simulink model "pole_placement_disturbance"  (R2017a)
settings: Solver=VariableStepAuto  StartTime=0.0  StopTime=10  RelTol=1e-3
values from neighbouring files (symbols this model uses):
  DCgain5 = D5d + C5cl*inv(eye(3)-A5cl)*B5d    [q13.m]    (also in q5.m; q5_reduced.m)
  h5 = 2.5*pi/w    [q13.m]    (also in q5.m = 2*pi/w; q5_reduced.m = 2*pi/w)
  K5_discr = place(A5d, B5d, P_discr)    [q13.m]    (also in q5.m; q5_reduced.m)
undefined symbols (not defined in the file or in its folder): A5d, B5d, C5d, D5d
settings Model: Creator=Aleksandra  LastModifiedBy=Aleksandra

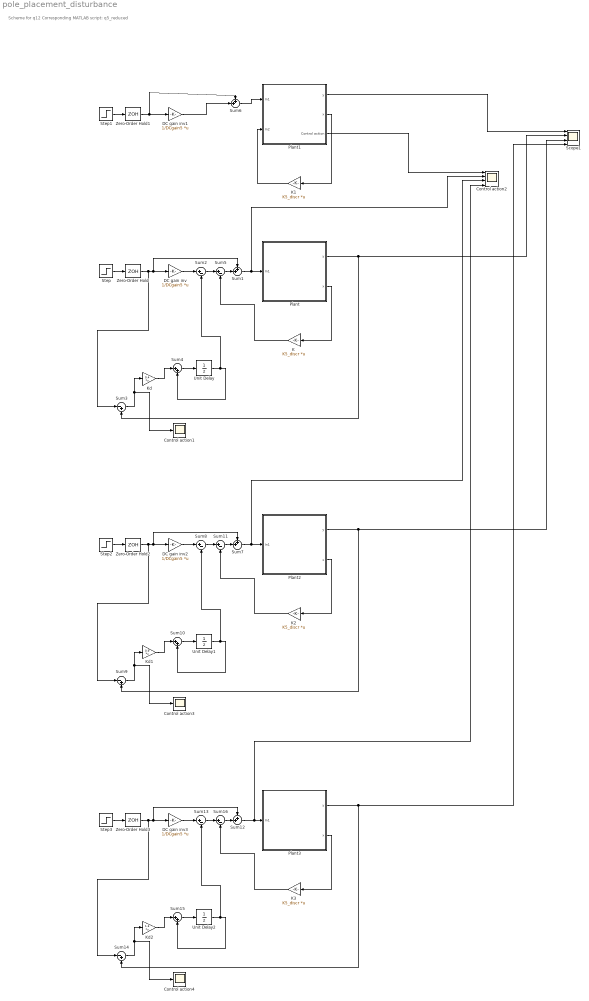
== system pole_placement_disturbance ==
  note: Scheme for q12
      | Corresponding MATLAB script: q5_reduced
  Control action1 : Scope
  Control action2 : Scope  NumInputPorts=4
  Control action3 : Scope
  Control action4 : Scope
  DC gain inv{,1..3} (4 alike) : Gain  Gain=1/DCgain5  Multiplication=Matrix(K*u)
  K{,1..3} (4 alike) : Gain  Gain=K5_discr  Multiplication=Matrix(K*u)
  Kd : Gain  Gain=0.4  Multiplication=Matrix(K*u)
  Kd1 : Gain  Gain=0.9  Multiplication=Matrix(K*u)
  Kd2 : Gain  Gain=1.3  Multiplication=Matrix(K*u)
  Plant : Subsystem
  Plant1 : Subsystem
  Plant2 : Subsystem
  Plant3 : Subsystem
  Scope1 : Scope  NumInputPorts=4
  Step{,1..3} (4 alike) : Step  Time=0  SampleTime=0
  Sum{1,6..7,12} (4 alike) : Sum  Inputs=++|
  Sum10 : Sum  Inputs=|++
  Sum{2,5,8,11,13,16} (6 alike) : Sum  Inputs=|+-
  Sum14 : Sum  Inputs=|-+
  Sum15 : Sum  Inputs=|++
  Sum3 : Sum  Inputs=|-+
  Sum4 : Sum  Inputs=|++
  Sum9 : Sum  Inputs=|-+
  Unit Delay : UnitDelay  SampleTime=-1
  Unit Delay1 : UnitDelay  SampleTime=-1
  Unit Delay2 : UnitDelay  SampleTime=-1
  Zero-Order Hold{,1..3} (4 alike) : ZeroOrderHold  SampleTime=h5
  wires:
  Step/1 -> Zero-Order Hold/1
  Plant/1(y) -> Sum3/2, Scope1/2
  Plant/2(x) -> K/1
  K/1 -> Sum5/2
  Zero-Order Hold/1 -> Sum3/1, Sum1/1, DC gain inv/1
  DC gain inv/1 -> Sum2/1
  Sum1/1 -> Control action2/2, Plant/1(In1)
  Sum2/1 -> Sum5/1
  Sum3/1 -> Control action1/1, Kd/1
  Sum4/1 -> Unit Delay/1
  Kd/1 -> Sum4/1
  Unit Delay/1 -> Sum2/2, Sum4/2
  Sum5/1 -> Sum1/2
  DC gain inv1/1 -> Sum6/2
  Plant1/3(Control action) -> Control action2/1
  Zero-Order Hold1/1 -> Sum6/1, DC gain inv1/1
  Plant1/1(y) -> Scope1/1
  K1/1 -> Plant1/2(In2)
  Plant1/2(x) -> K1/1
  Step1/1 -> Zero-Order Hold1/1
  Sum6/1 -> Plant1/1(In1)
  Zero-Order Hold2/1 -> Sum9/1, Sum7/1, DC gain inv2/1
  Plant2/1(y) -> Scope1/3, Sum9/2
  Step2/1 -> Zero-Order Hold2/1
  Sum10/1 -> Unit Delay1/1
  Sum11/1 -> Sum7/2
  Unit Delay1/1 -> Sum8/2, Sum10/2
  Sum7/1 -> Control action2/3, Plant2/1(In1)
  Plant2/2(x) -> K2/1
  Sum8/1 -> Sum11/1
  Kd1/1 -> Sum10/1
  K2/1 -> Sum11/2
  Sum9/1 -> Control action3/1, Kd1/1
  DC gain inv2/1 -> Sum8/1
  Zero-Order Hold3/1 -> Sum14/1, Sum12/1, DC gain inv3/1
  Plant3/1(y) -> Scope1/4, Sum14/2
  Step3/1 -> Zero-Order Hold3/1
  Sum15/1 -> Unit Delay2/1
  Sum16/1 -> Sum12/2
  Unit Delay2/1 -> Sum13/2, Sum15/2
  Sum12/1 -> Control action2/4, Plant3/1(In1)
  Plant3/2(x) -> K3/1
  Sum13/1 -> Sum16/1
  Kd2/1 -> Sum15/1
  K3/1 -> Sum16/2
  Sum14/1 -> Control action4/1, Kd2/1
  DC gain inv3/1 -> Sum13/1

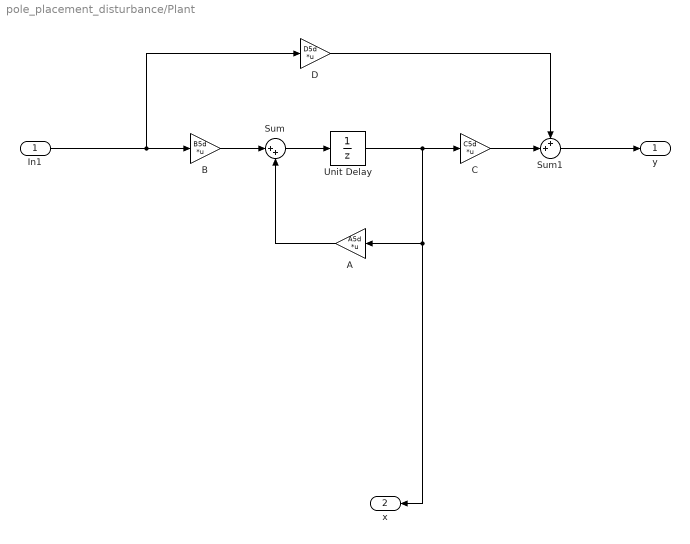
== system pole_placement_disturbance/Plant ==
  In1 : Inport
  A : Gain  Gain=A5d  Multiplication=Matrix(K*u)
  B : Gain  Gain=B5d  Multiplication=Matrix(K*u)
  C : Gain  Gain=C5d  Multiplication=Matrix(K*u)
  D : Gain  Gain=D5d  Multiplication=Matrix(K*u)
  Sum : Sum  Inputs=|++
  Sum1 : Sum  Inputs=++|
  Unit Delay : UnitDelay  SampleTime=-1
  y : Outport
  x : Outport  Port=2
  wires:
  Sum/1 -> Unit Delay/1
  A/1 -> Sum/2
  D/1 -> Sum1/1
  C/1 -> Sum1/2
  Sum1/1 -> y/1
  B/1 -> Sum/1
  In1/1 -> D/1, B/1
  Unit Delay/1 -> x/1, A/1, C/1

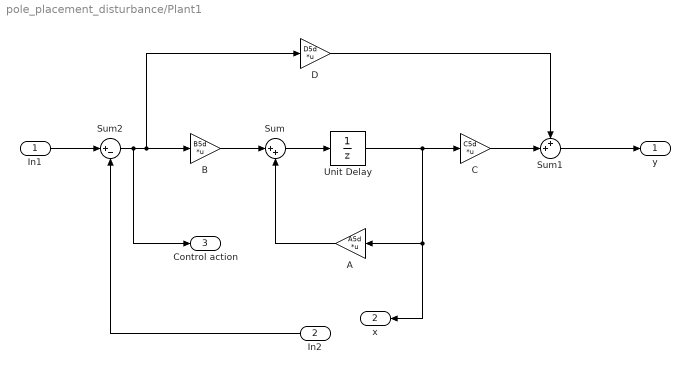
== system pole_placement_disturbance/Plant1 ==
  In1 : Inport
  In2 : Inport  Port=2
  A : Gain  Gain=A5d  Multiplication=Matrix(K*u)
  B : Gain  Gain=B5d  Multiplication=Matrix(K*u)
  C : Gain  Gain=C5d  Multiplication=Matrix(K*u)
  D : Gain  Gain=D5d  Multiplication=Matrix(K*u)
  Sum : Sum  Inputs=|++
  Sum1 : Sum  Inputs=++|
  Sum2 : Sum  Inputs=|+-
  Unit Delay : UnitDelay  SampleTime=-1
  y : Outport
  x : Outport  Port=2
  Control action : Outport  Port=3
  wires:
  Sum/1 -> Unit Delay/1
  A/1 -> Sum/2
  D/1 -> Sum1/1
  C/1 -> Sum1/2
  Sum1/1 -> y/1
  B/1 -> Sum/1
  Sum2/1 -> Control action/1, D/1, B/1
  Unit Delay/1 -> x/1, A/1, C/1
  In2/1 -> Sum2/2
  In1/1 -> Sum2/1

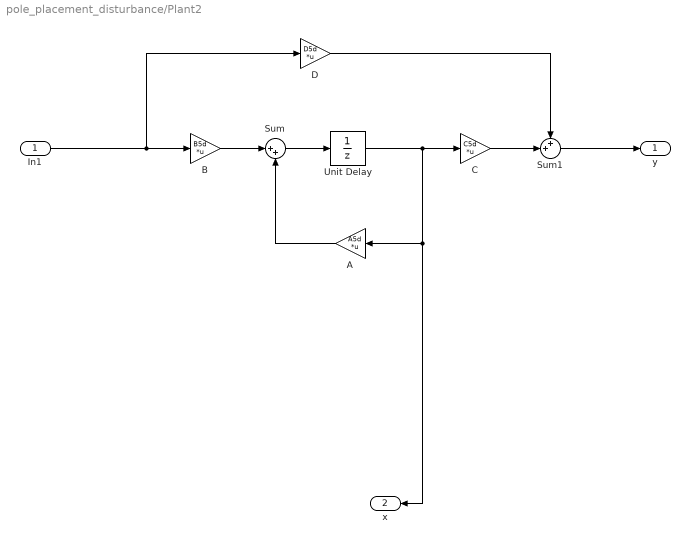
== system pole_placement_disturbance/Plant2 ==
  In1 : Inport
  A : Gain  Gain=A5d  Multiplication=Matrix(K*u)
  B : Gain  Gain=B5d  Multiplication=Matrix(K*u)
  C : Gain  Gain=C5d  Multiplication=Matrix(K*u)
  D : Gain  Gain=D5d  Multiplication=Matrix(K*u)
  Sum : Sum  Inputs=|++
  Sum1 : Sum  Inputs=++|
  Unit Delay : UnitDelay  SampleTime=-1
  y : Outport
  x : Outport  Port=2
  wires:
  Sum/1 -> Unit Delay/1
  A/1 -> Sum/2
  D/1 -> Sum1/1
  C/1 -> Sum1/2
  Sum1/1 -> y/1
  B/1 -> Sum/1
  In1/1 -> D/1, B/1
  Unit Delay/1 -> x/1, A/1, C/1

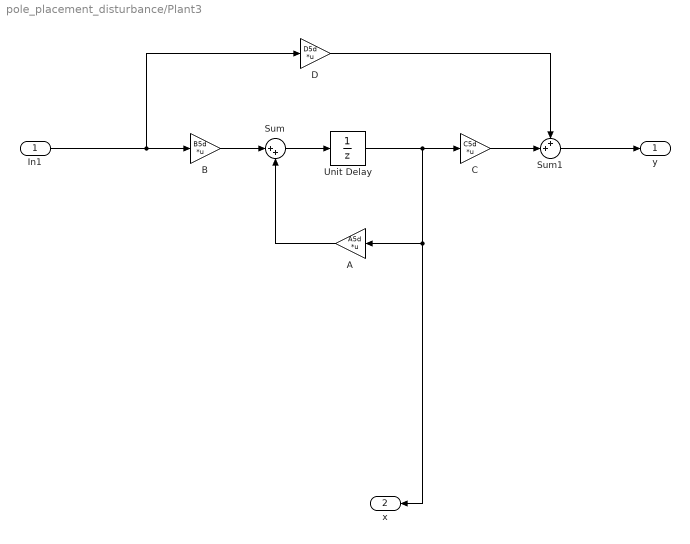
== system pole_placement_disturbance/Plant3 ==
  In1 : Inport
  A : Gain  Gain=A5d  Multiplication=Matrix(K*u)
  B : Gain  Gain=B5d  Multiplication=Matrix(K*u)
  C : Gain  Gain=C5d  Multiplication=Matrix(K*u)
  D : Gain  Gain=D5d  Multiplication=Matrix(K*u)
  Sum : Sum  Inputs=|++
  Sum1 : Sum  Inputs=++|
  Unit Delay : UnitDelay  SampleTime=-1
  y : Outport
  x : Outport  Port=2
  wires:
  Sum/1 -> Unit Delay/1
  A/1 -> Sum/2
  D/1 -> Sum1/1
  C/1 -> Sum1/2
  Sum1/1 -> y/1
  B/1 -> Sum/1
  In1/1 -> D/1, B/1
  Unit Delay/1 -> x/1, A/1, C/1
